simulink model "CryoDetMultiChan_CMB"  (R2016b)
settings: Solver=ode45  StartTime=0.0  StopTime=1000e-6  MaxStep=Tclk/4  RelTol=1e-3
values from neighbouring files (symbols this model uses):
  ds_axi = 16    [setupCryoFPGA_CMB.m]
  Fclk = Fadc    (= 307200000)    [setupCryoFPGA.m]    (also in setupCryoFPGA_CMB.m; setupCryoFPGAorig.m = 312500000)
  notch = tf( [1 a*wNotch/Q wNotch^2], [1 wNotch/Q wNotch^2])    [setupCryoFPGA.m]    (also in setupCryoFPGA_CMB.m; setupCryoFPGAorig.m)
  notch2 = tf( [1 a*wNotch/Q wNotch^2], [1 wNotch/Q wNotch^2])    [setupCryoFPGA.m]    (also in setupCryoFPGA_CMB.m; setupCryoFPGAorig.m)
  notch3 = tf( [1 a*wNotch/Q wNotch^2], [1 wNotch/Q wNotch^2])    [setupCryoFPGA.m]    (also in setupCryoFPGA_CMB.m; setupCryoFPGAorig.m)
  notch4 = tf( [1 a*wNotch/Q wNotch^2], [1 wNotch/Q wNotch^2])    [setupCryoFPGA.m]    (also in setupCryoFPGA_CMB.m; setupCryoFPGAorig.m)
  Tclk = 1/Fclk    (= 3.25520833333e-09)    [setupCryoFPGA.m]    (also in setupCryoFPGA_CMB.m; setupCryoFPGAorig.m = 3.2e-09)
  Ts = 1/Fadc    (= 3.25520833333e-09)    [setupCryoFPGA.m]    (also in setupCryoFPGA_CMB.m; setupCryoFPGAorig.m = 3.2e-09)
undefined symbols (not defined in the file or in its folder): AXI4, i, Lite, xlipgetpartsetting
libraries: xbsIndex_r4 x2077, CryoDetLib x32, hdlsllib x6, simulink x3
(part 4 of 15)

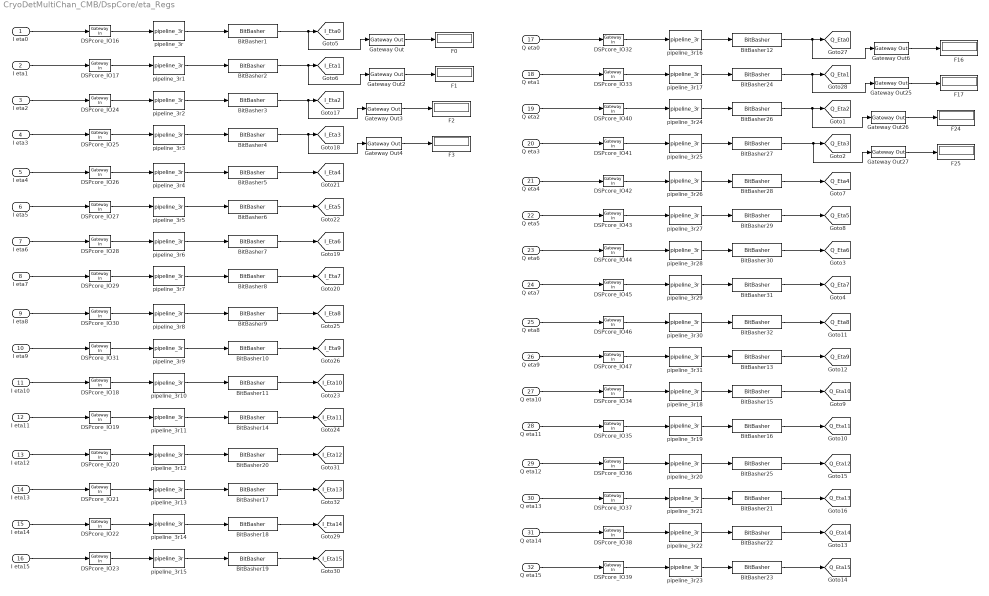
== system CryoDetMultiChan_CMB/DspCore/eta_Regs ==
  "I eta0 " : Inport
  I eta1 : Inport  Port=2
  I eta2 : Inport  Port=3
  I eta3 : Inport  Port=4
  I eta4 : Inport  Port=5
  I eta5 : Inport  Port=6
  I eta6 : Inport  Port=7
  I eta7 : Inport  Port=8
  I eta8 : Inport  Port=9
  I eta9 : Inport  Port=10
  I eta10 : Inport  Port=11
  I eta11 : Inport  Port=12
  I eta12 : Inport  Port=13
  I eta13 : Inport  Port=14
  I eta14 : Inport  Port=15
  I eta15 : Inport  Port=16
  Q eta0 : Inport  Port=17
  Q eta1 : Inport  Port=18
  Q eta2 : Inport  Port=19
  Q eta3 : Inport  Port=20
  Q eta4 : Inport  Port=21
  Q eta5 : Inport  Port=22
  Q eta6 : Inport  Port=23
  Q eta7 : Inport  Port=24
  Q eta8 : Inport  Port=25
  Q eta9 : Inport  Port=26
  Q eta10 : Inport  Port=27
  Q eta11 : Inport  Port=28
  Q eta12 : Inport  Port=29
  Q eta13 : Inport  Port=30
  Q eta14 : Inport  Port=31
  Q eta15 : Inport  Port=32
  BitBasher{1..32} (32 alike) : xbsIndex_r4/BitBasher  bitexpr=a={b[24:0]}  display_expr=on  sr_1=a  arith_type1=Unsigned  bin_pt1=0  sr_2=2  arith_type2=Unsigned  bin_pt2=0  sr_3=3  arith_type3=Unsigned  bin_pt3=0  sr_4=4  arith_type4=Unsigned  bin_pt4=0  dbl_ovrd=off  block_type=bitbasher
  DSPcore_IO16 : xbsIndex_r4/Gateway In  gui_display_data_type=Fixed-point  arith_type="Signed  (2's comp)"  n_bits=32  bin_pt=0  preci_type=Single  exp_width=8  frac_width=24  rows=1  columns=1  quantization=Truncate  overflow=Wrap  period=Tclk*ds_axi  UseAsADC=off  ADCChannel='1'  interface=AXI4-Lite  automatic_assignment=off  address_offset=hex2dec('A00')  intf_name=''  intf_description=''  default_value=0  timing_constraint=None  locs_specified=off  LOCs={}  io_standard={}  inherit_from_input=off  hdl_port=on  dbl_ovrd=off  block_type=gatewayin
  DSPcore_IO17 : xbsIndex_r4/Gateway In  gui_display_data_type=Fixed-point  arith_type="Signed  (2's comp)"  n_bits=32  bin_pt=0  preci_type=Single  exp_width=8  frac_width=24  rows=1  columns=1  quantization=Truncate  overflow=Wrap  period=Tclk*ds_axi  UseAsADC=off  ADCChannel='1'  interface=AXI4-Lite  automatic_assignment=off  address_offset=hex2dec('A08')  intf_name=''  intf_description=''  default_value=0  timing_constraint=None  locs_specified=off  LOCs={}  io_standard={}  inherit_from_input=off  hdl_port=on  dbl_ovrd=off  block_type=gatewayin
  DSPcore_IO18 : xbsIndex_r4/Gateway In  gui_display_data_type=Fixed-point  arith_type="Signed  (2's comp)"  n_bits=32  bin_pt=0  preci_type=Single  exp_width=8  frac_width=24  rows=1  columns=1  quantization=Truncate  overflow=Wrap  period=Tclk*ds_axi  UseAsADC=off  ADCChannel='1'  interface=AXI4-Lite  automatic_assignment=off  address_offset=hex2dec('A50')  intf_name=''  intf_description=''  default_value=0  timing_constraint=None  locs_specified=off  LOCs={}  io_standard={}  inherit_from_input=off  hdl_port=on  dbl_ovrd=off  block_type=gatewayin
  DSPcore_IO19 : xbsIndex_r4/Gateway In  gui_display_data_type=Fixed-point  arith_type="Signed  (2's comp)"  n_bits=32  bin_pt=0  preci_type=Single  exp_width=8  frac_width=24  rows=1  columns=1  quantization=Truncate  overflow=Wrap  period=Tclk*ds_axi  UseAsADC=off  ADCChannel='1'  interface=AXI4-Lite  automatic_assignment=off  address_offset=hex2dec('A58')  intf_name=''  intf_description=''  default_value=0  timing_constraint=None  locs_specified=off  LOCs={}  io_standard={}  inherit_from_input=off  hdl_port=on  dbl_ovrd=off  block_type=gatewayin
  DSPcore_IO20 : xbsIndex_r4/Gateway In  gui_display_data_type=Fixed-point  arith_type="Signed  (2's comp)"  n_bits=32  bin_pt=0  preci_type=Single  exp_width=8  frac_width=24  rows=1  columns=1  quantization=Truncate  overflow=Wrap  period=Tclk*ds_axi  UseAsADC=off  ADCChannel='1'  interface=AXI4-Lite  automatic_assignment=off  address_offset=hex2dec('A60')  intf_name=''  intf_description=''  default_value=0  timing_constraint=None  locs_specified=off  LOCs={}  io_standard={}  inherit_from_input=off  hdl_port=on  dbl_ovrd=off  block_type=gatewayin
  DSPcore_IO21 : xbsIndex_r4/Gateway In  gui_display_data_type=Fixed-point  arith_type="Signed  (2's comp)"  n_bits=32  bin_pt=0  preci_type=Single  exp_width=8  frac_width=24  rows=1  columns=1  quantization=Truncate  overflow=Wrap  period=Tclk*ds_axi  UseAsADC=off  ADCChannel='1'  interface=AXI4-Lite  automatic_assignment=off  address_offset=hex2dec('A68')  intf_name=''  intf_description=''  default_value=0  timing_constraint=None  locs_specified=off  LOCs={}  io_standard={}  inherit_from_input=off  hdl_port=on  dbl_ovrd=off  block_type=gatewayin
  DSPcore_IO22 : xbsIndex_r4/Gateway In  gui_display_data_type=Fixed-point  arith_type="Signed  (2's comp)"  n_bits=32  bin_pt=0  preci_type=Single  exp_width=8  frac_width=24  rows=1  columns=1  quantization=Truncate  overflow=Wrap  period=Tclk*ds_axi  UseAsADC=off  ADCChannel='1'  interface=AXI4-Lite  automatic_assignment=off  address_offset=hex2dec('A70')  intf_name=''  intf_description=''  default_value=0  timing_constraint=None  locs_specified=off  LOCs={}  io_standard={}  inherit_from_input=off  hdl_port=on  dbl_ovrd=off  block_type=gatewayin
  DSPcore_IO23 : xbsIndex_r4/Gateway In  gui_display_data_type=Fixed-point  arith_type="Signed  (2's comp)"  n_bits=32  bin_pt=0  preci_type=Single  exp_width=8  frac_width=24  rows=1  columns=1  quantization=Truncate  overflow=Wrap  period=Tclk*ds_axi  UseAsADC=off  ADCChannel='1'  interface=AXI4-Lite  automatic_assignment=off  address_offset=hex2dec('A78')  intf_name=''  intf_description=''  default_value=0  timing_constraint=None  locs_specified=off  LOCs={}  io_standard={}  inherit_from_input=off  hdl_port=on  dbl_ovrd=off  block_type=gatewayin
  DSPcore_IO24 : xbsIndex_r4/Gateway In  gui_display_data_type=Fixed-point  arith_type="Signed  (2's comp)"  n_bits=32  bin_pt=0  preci_type=Single  exp_width=8  frac_width=24  rows=1  columns=1  quantization=Truncate  overflow=Wrap  period=Tclk*ds_axi  UseAsADC=off  ADCChannel='1'  interface=AXI4-Lite  automatic_assignment=off  address_offset=hex2dec('A10')  intf_name=''  intf_description=''  default_value=0  timing_constraint=None  locs_specified=off  LOCs={}  io_standard={}  inherit_from_input=off  hdl_port=on  dbl_ovrd=off  block_type=gatewayin
  DSPcore_IO25 : xbsIndex_r4/Gateway In  gui_display_data_type=Fixed-point  arith_type="Signed  (2's comp)"  n_bits=32  bin_pt=0  preci_type=Single  exp_width=8  frac_width=24  rows=1  columns=1  quantization=Truncate  overflow=Wrap  period=Tclk*ds_axi  UseAsADC=off  ADCChannel='1'  interface=AXI4-Lite  automatic_assignment=off  address_offset=hex2dec('A18')  intf_name=''  intf_description=''  default_value=0  timing_constraint=None  locs_specified=off  LOCs={}  io_standard={}  inherit_from_input=off  hdl_port=on  dbl_ovrd=off  block_type=gatewayin
  DSPcore_IO26 : xbsIndex_r4/Gateway In  gui_display_data_type=Fixed-point  arith_type="Signed  (2's comp)"  n_bits=32  bin_pt=0  preci_type=Single  exp_width=8  frac_width=24  rows=1  columns=1  quantization=Truncate  overflow=Wrap  period=Tclk*ds_axi  UseAsADC=off  ADCChannel='1'  interface=AXI4-Lite  automatic_assignment=off  address_offset=hex2dec('A20')  intf_name=''  intf_description=''  default_value=0  timing_constraint=None  locs_specified=off  LOCs={}  io_standard={}  inherit_from_input=off  hdl_port=on  dbl_ovrd=off  block_type=gatewayin
  DSPcore_IO27 : xbsIndex_r4/Gateway In  gui_display_data_type=Fixed-point  arith_type="Signed  (2's comp)"  n_bits=32  bin_pt=0  preci_type=Single  exp_width=8  frac_width=24  rows=1  columns=1  quantization=Truncate  overflow=Wrap  period=Tclk*ds_axi  UseAsADC=off  ADCChannel='1'  interface=AXI4-Lite  automatic_assignment=off  address_offset=hex2dec('A28')  intf_name=''  intf_description=''  default_value=0  timing_constraint=None  locs_specified=off  LOCs={}  io_standard={}  inherit_from_input=off  hdl_port=on  dbl_ovrd=off  block_type=gatewayin
  DSPcore_IO28 : xbsIndex_r4/Gateway In  gui_display_data_type=Fixed-point  arith_type="Signed  (2's comp)"  n_bits=32  bin_pt=0  preci_type=Single  exp_width=8  frac_width=24  rows=1  columns=1  quantization=Truncate  overflow=Wrap  period=Tclk*ds_axi  UseAsADC=off  ADCChannel='1'  interface=AXI4-Lite  automatic_assignment=off  address_offset=hex2dec('A30')  intf_name=''  intf_description=''  default_value=0  timing_constraint=None  locs_specified=off  LOCs={}  io_standard={}  inherit_from_input=off  hdl_port=on  dbl_ovrd=off  block_type=gatewayin
  DSPcore_IO29 : xbsIndex_r4/Gateway In  gui_display_data_type=Fixed-point  arith_type="Signed  (2's comp)"  n_bits=32  bin_pt=0  preci_type=Single  exp_width=8  frac_width=24  rows=1  columns=1  quantization=Truncate  overflow=Wrap  period=Tclk*ds_axi  UseAsADC=off  ADCChannel='1'  interface=AXI4-Lite  automatic_assignment=off  address_offset=hex2dec('A38')  intf_name=''  intf_description=''  default_value=0  timing_constraint=None  locs_specified=off  LOCs={}  io_standard={}  inherit_from_input=off  hdl_port=on  dbl_ovrd=off  block_type=gatewayin
  DSPcore_IO30 : xbsIndex_r4/Gateway In  gui_display_data_type=Fixed-point  arith_type="Signed  (2's comp)"  n_bits=32  bin_pt=0  preci_type=Single  exp_width=8  frac_width=24  rows=1  columns=1  quantization=Truncate  overflow=Wrap  period=Tclk*ds_axi  UseAsADC=off  ADCChannel='1'  interface=AXI4-Lite  automatic_assignment=off  address_offset=hex2dec('A40')  intf_name=''  intf_description=''  default_value=0  timing_constraint=None  locs_specified=off  LOCs={}  io_standard={}  inherit_from_input=off  hdl_port=on  dbl_ovrd=off  block_type=gatewayin
  DSPcore_IO31 : xbsIndex_r4/Gateway In  gui_display_data_type=Fixed-point  arith_type="Signed  (2's comp)"  n_bits=32  bin_pt=0  preci_type=Single  exp_width=8  frac_width=24  rows=1  columns=1  quantization=Truncate  overflow=Wrap  period=Tclk*ds_axi  UseAsADC=off  ADCChannel='1'  interface=AXI4-Lite  automatic_assignment=off  address_offset=hex2dec('A48')  intf_name=''  intf_description=''  default_value=0  timing_constraint=None  locs_specified=off  LOCs={}  io_standard={}  inherit_from_input=off  hdl_port=on  dbl_ovrd=off  block_type=gatewayin
  DSPcore_IO32 : xbsIndex_r4/Gateway In  gui_display_data_type=Fixed-point  arith_type="Signed  (2's comp)"  n_bits=32  bin_pt=0  preci_type=Single  exp_width=8  frac_width=24  rows=1  columns=1  quantization=Truncate  overflow=Wrap  period=Tclk*ds_axi  UseAsADC=off  ADCChannel='1'  interface=AXI4-Lite  automatic_assignment=off  address_offset=hex2dec('A04')  intf_name=''  intf_description=''  default_value=0  timing_constraint=None  locs_specified=off  LOCs={}  io_standard={}  inherit_from_input=off  hdl_port=on  dbl_ovrd=off  block_type=gatewayin
  DSPcore_IO33 : xbsIndex_r4/Gateway In  gui_display_data_type=Fixed-point  arith_type="Signed  (2's comp)"  n_bits=32  bin_pt=0  preci_type=Single  exp_width=8  frac_width=24  rows=1  columns=1  quantization=Truncate  overflow=Wrap  period=Tclk*ds_axi  UseAsADC=off  ADCChannel='1'  interface=AXI4-Lite  automatic_assignment=off  address_offset=hex2dec('A0C')  intf_name=''  intf_description=''  default_value=0  timing_constraint=None  locs_specified=off  LOCs={}  io_standard={}  inherit_from_input=off  hdl_port=on  dbl_ovrd=off  block_type=gatewayin
  DSPcore_IO34 : xbsIndex_r4/Gateway In  gui_display_data_type=Fixed-point  arith_type="Signed  (2's comp)"  n_bits=32  bin_pt=0  preci_type=Single  exp_width=8  frac_width=24  rows=1  columns=1  quantization=Truncate  overflow=Wrap  period=Tclk*ds_axi  UseAsADC=off  ADCChannel='1'  interface=AXI4-Lite  automatic_assignment=off  address_offset=hex2dec('A54')  intf_name=''  intf_description=''  default_value=0  timing_constraint=None  locs_specified=off  LOCs={}  io_standard={}  inherit_from_input=off  hdl_port=on  dbl_ovrd=off  block_type=gatewayin
  DSPcore_IO35 : xbsIndex_r4/Gateway In  gui_display_data_type=Fixed-point  arith_type="Signed  (2's comp)"  n_bits=32  bin_pt=0  preci_type=Single  exp_width=8  frac_width=24  rows=1  columns=1  quantization=Truncate  overflow=Wrap  period=Tclk*ds_axi  UseAsADC=off  ADCChannel='1'  interface=AXI4-Lite  automatic_assignment=off  address_offset=hex2dec('A5C')  intf_name=''  intf_description=''  default_value=0  timing_constraint=None  locs_specified=off  LOCs={}  io_standard={}  inherit_from_input=off  hdl_port=on  dbl_ovrd=off  block_type=gatewayin
  DSPcore_IO36 : xbsIndex_r4/Gateway In  gui_display_data_type=Fixed-point  arith_type="Signed  (2's comp)"  n_bits=32  bin_pt=0  preci_type=Single  exp_width=8  frac_width=24  rows=1  columns=1  quantization=Truncate  overflow=Wrap  period=Tclk*ds_axi  UseAsADC=off  ADCChannel='1'  interface=AXI4-Lite  automatic_assignment=off  address_offset=hex2dec('A64')  intf_name=''  intf_description=''  default_value=0  timing_constraint=None  locs_specified=off  LOCs={}  io_standard={}  inherit_from_input=off  hdl_port=on  dbl_ovrd=off  block_type=gatewayin
  DSPcore_IO37 : xbsIndex_r4/Gateway In  gui_display_data_type=Fixed-point  arith_type="Signed  (2's comp)"  n_bits=32  bin_pt=0  preci_type=Single  exp_width=8  frac_width=24  rows=1  columns=1  quantization=Truncate  overflow=Wrap  period=Tclk*ds_axi  UseAsADC=off  ADCChannel='1'  interface=AXI4-Lite  automatic_assignment=off  address_offset=hex2dec('A6C')  intf_name=''  intf_description=''  default_value=0  timing_constraint=None  locs_specified=off  LOCs={}  io_standard={}  inherit_from_input=off  hdl_port=on  dbl_ovrd=off  block_type=gatewayin
  DSPcore_IO38 : xbsIndex_r4/Gateway In  gui_display_data_type=Fixed-point  arith_type="Signed  (2's comp)"  n_bits=32  bin_pt=0  preci_type=Single  exp_width=8  frac_width=24  rows=1  columns=1  quantization=Truncate  overflow=Wrap  period=Tclk*ds_axi  UseAsADC=off  ADCChannel='1'  interface=AXI4-Lite  automatic_assignment=off  address_offset=hex2dec('A74')  intf_name=''  intf_description=''  default_value=0  timing_constraint=None  locs_specified=off  LOCs={}  io_standard={}  inherit_from_input=off  hdl_port=on  dbl_ovrd=off  block_type=gatewayin
  DSPcore_IO39 : xbsIndex_r4/Gateway In  gui_display_data_type=Fixed-point  arith_type="Signed  (2's comp)"  n_bits=32  bin_pt=0  preci_type=Single  exp_width=8  frac_width=24  rows=1  columns=1  quantization=Truncate  overflow=Wrap  period=Tclk*ds_axi  UseAsADC=off  ADCChannel='1'  interface=AXI4-Lite  automatic_assignment=off  address_offset=hex2dec('A7C')  intf_name=''  intf_description=''  default_value=0  timing_constraint=None  locs_specified=off  LOCs={}  io_standard={}  inherit_from_input=off  hdl_port=on  dbl_ovrd=off  block_type=gatewayin
  DSPcore_IO40 : xbsIndex_r4/Gateway In  gui_display_data_type=Fixed-point  arith_type="Signed  (2's comp)"  n_bits=32  bin_pt=0  preci_type=Single  exp_width=8  frac_width=24  rows=1  columns=1  quantization=Truncate  overflow=Wrap  period=Tclk*ds_axi  UseAsADC=off  ADCChannel='1'  interface=AXI4-Lite  automatic_assignment=off  address_offset=hex2dec('A14')  intf_name=''  intf_description=''  default_value=0  timing_constraint=None  locs_specified=off  LOCs={}  io_standard={}  inherit_from_input=off  hdl_port=on  dbl_ovrd=off  block_type=gatewayin
  DSPcore_IO41 : xbsIndex_r4/Gateway In  gui_display_data_type=Fixed-point  arith_type="Signed  (2's comp)"  n_bits=32  bin_pt=0  preci_type=Single  exp_width=8  frac_width=24  rows=1  columns=1  quantization=Truncate  overflow=Wrap  period=Tclk*ds_axi  UseAsADC=off  ADCChannel='1'  interface=AXI4-Lite  automatic_assignment=off  address_offset=hex2dec('A1C')  intf_name=''  intf_description=''  default_value=0  timing_constraint=None  locs_specified=off  LOCs={}  io_standard={}  inherit_from_input=off  hdl_port=on  dbl_ovrd=off  block_type=gatewayin
  DSPcore_IO42 : xbsIndex_r4/Gateway In  gui_display_data_type=Fixed-point  arith_type="Signed  (2's comp)"  n_bits=32  bin_pt=0  preci_type=Single  exp_width=8  frac_width=24  rows=1  columns=1  quantization=Truncate  overflow=Wrap  period=Tclk*ds_axi  UseAsADC=off  ADCChannel='1'  interface=AXI4-Lite  automatic_assignment=off  address_offset=hex2dec('A24')  intf_name=''  intf_description=''  default_value=0  timing_constraint=None  locs_specified=off  LOCs={}  io_standard={}  inherit_from_input=off  hdl_port=on  dbl_ovrd=off  block_type=gatewayin
  DSPcore_IO43 : xbsIndex_r4/Gateway In  gui_display_data_type=Fixed-point  arith_type="Signed  (2's comp)"  n_bits=32  bin_pt=0  preci_type=Single  exp_width=8  frac_width=24  rows=1  columns=1  quantization=Truncate  overflow=Wrap  period=Tclk*ds_axi  UseAsADC=off  ADCChannel='1'  interface=AXI4-Lite  automatic_assignment=off  address_offset=hex2dec('A2C')  intf_name=''  intf_description=''  default_value=0  timing_constraint=None  locs_specified=off  LOCs={}  io_standard={}  inherit_from_input=off  hdl_port=on  dbl_ovrd=off  block_type=gatewayin
  DSPcore_IO44 : xbsIndex_r4/Gateway In  gui_display_data_type=Fixed-point  arith_type="Signed  (2's comp)"  n_bits=32  bin_pt=0  preci_type=Single  exp_width=8  frac_width=24  rows=1  columns=1  quantization=Truncate  overflow=Wrap  period=Tclk*ds_axi  UseAsADC=off  ADCChannel='1'  interface=AXI4-Lite  automatic_assignment=off  address_offset=hex2dec('A34')  intf_name=''  intf_description=''  default_value=0  timing_constraint=None  locs_specified=off  LOCs={}  io_standard={}  inherit_from_input=off  hdl_port=on  dbl_ovrd=off  block_type=gatewayin
  DSPcore_IO45 : xbsIndex_r4/Gateway In  gui_display_data_type=Fixed-point  arith_type="Signed  (2's comp)"  n_bits=32  bin_pt=0  preci_type=Single  exp_width=8  frac_width=24  rows=1  columns=1  quantization=Truncate  overflow=Wrap  period=Tclk*ds_axi  UseAsADC=off  ADCChannel='1'  interface=AXI4-Lite  automatic_assignment=off  address_offset=hex2dec('A3C')  intf_name=''  intf_description=''  default_value=0  timing_constraint=None  locs_specified=off  LOCs={}  io_standard={}  inherit_from_input=off  hdl_port=on  dbl_ovrd=off  block_type=gatewayin
  DSPcore_IO46 : xbsIndex_r4/Gateway In  gui_display_data_type=Fixed-point  arith_type="Signed  (2's comp)"  n_bits=32  bin_pt=0  preci_type=Single  exp_width=8  frac_width=24  rows=1  columns=1  quantization=Truncate  overflow=Wrap  period=Tclk*ds_axi  UseAsADC=off  ADCChannel='1'  interface=AXI4-Lite  automatic_assignment=off  address_offset=hex2dec('A44')  intf_name=''  intf_description=''  default_value=0  timing_constraint=None  locs_specified=off  LOCs={}  io_standard={}  inherit_from_input=off  hdl_port=on  dbl_ovrd=off  block_type=gatewayin
  DSPcore_IO47 : xbsIndex_r4/Gateway In  gui_display_data_type=Fixed-point  arith_type="Signed  (2's comp)"  n_bits=32  bin_pt=0  preci_type=Single  exp_width=8  frac_width=24  rows=1  columns=1  quantization=Truncate  overflow=Wrap  period=Tclk*ds_axi  UseAsADC=off  ADCChannel='1'  interface=AXI4-Lite  automatic_assignment=off  address_offset=hex2dec('A4C')  intf_name=''  intf_description=''  default_value=0  timing_constraint=None  locs_specified=off  LOCs={}  io_standard={}  inherit_from_input=off  hdl_port=on  dbl_ovrd=off  block_type=gatewayin
  F{0..3,16..17,24..25} (8 alike) : Display
  Gateway Out{,2..4,6,25..27} (8 alike) : xbsIndex_r4/Gateway Out  inherit_from_input=on  hdl_port=off  rows=1  columns=1  UseAsDAC=off  DACChannel='1'  interface=None  automatic_assignment=on  address_offset=hex2dec('00')  intf_name=''  intf_description=''  timing_constraint=None  locs_specified=off  LOCs={}  io_standard={}  block_type=gatewayout
  pipeline_3r{,1..31} (32 alike) : CryoDetLib/pipeline_3r
  tag scope: I_Eta0=global, I_Eta10=global, I_Eta11=global, I_Eta12=global, I_Eta13=global, I_Eta14=global, I_Eta15=global, I_Eta1=global, I_Eta2=global, I_Eta3=global, I_Eta4=global, I_Eta5=global, I_Eta6=global, I_Eta7=global, I_Eta8=global, I_Eta9=global, Q_Eta0=global, Q_Eta10=global, Q_Eta11=global, Q_Eta12=global, Q_Eta13=global, Q_Eta14=global, Q_Eta15=global, Q_Eta1=global, Q_Eta2=global, Q_Eta3=global, Q_Eta4=global, Q_Eta5=global, Q_Eta6=global, Q_Eta7=global, Q_Eta8=global, Q_Eta9=global
  wires:
  I eta14/1 -> DSPcore_IO22/1
  BitBasher5/1 -> [I_Eta4]
  DSPcore_IO26/1 -> pipeline_3r4/1
  BitBasher17/1 -> [I_Eta13]
  I eta13/1 -> DSPcore_IO21/1
  DSPcore_IO27/1 -> pipeline_3r5/1
  I eta15/1 -> DSPcore_IO23/1
  BitBasher11/1 -> [I_Eta10]
  I eta7/1 -> DSPcore_IO29/1
  I eta11/1 -> DSPcore_IO19/1
  I eta9/1 -> DSPcore_IO31/1
  Gateway Out4/1 -> F3/1
  BitBasher4/1 -> [I_Eta3], Gateway Out4/1
  I eta5/1 -> DSPcore_IO27/1
  DSPcore_IO23/1 -> pipeline_3r15/1
  DSPcore_IO21/1 -> pipeline_3r13/1
  DSPcore_IO31/1 -> pipeline_3r9/1
  BitBasher6/1 -> [I_Eta5]
  I eta8/1 -> DSPcore_IO30/1
  DSPcore_IO20/1 -> pipeline_3r12/1
  BitBasher20/1 -> [I_Eta12]
  DSPcore_IO25/1 -> pipeline_3r3/1
  I eta4/1 -> DSPcore_IO26/1
  Gateway Out2/1 -> F1/1
  BitBasher2/1 -> [I_Eta1], Gateway Out2/1
  DSPcore_IO30/1 -> pipeline_3r8/1
  BitBasher14/1 -> [I_Eta11]
  BitBasher19/1 -> [I_Eta15]
  I eta10/1 -> DSPcore_IO18/1
  BitBasher10/1 -> [I_Eta9]
  DSPcore_IO19/1 -> pipeline_3r11/1
  DSPcore_IO24/1 -> pipeline_3r2/1
  I eta2/1 -> DSPcore_IO24/1
  Gateway Out3/1 -> F2/1
  BitBasher3/1 -> [I_Eta2], Gateway Out3/1
  DSPcore_IO22/1 -> pipeline_3r14/1
  DSPcore_IO17/1 -> pipeline_3r1/1
  I eta1/1 -> DSPcore_IO17/1
  BitBasher9/1 -> [I_Eta8]
  DSPcore_IO29/1 -> pipeline_3r7/1
  BitBasher18/1 -> [I_Eta14]
  DSPcore_IO18/1 -> pipeline_3r10/1
  I eta6/1 -> DSPcore_IO28/1
  I eta3/1 -> DSPcore_IO25/1
  "I eta0 "/1 -> DSPcore_IO16/1
  Gateway Out/1 -> F0/1
  BitBasher1/1 -> [I_Eta0], Gateway Out/1
  DSPcore_IO16/1 -> pipeline_3r/1
  pipeline_3r/1 -> BitBasher1/1
  BitBasher7/1 -> [I_Eta6]
  BitBasher8/1 -> [I_Eta7]
  I eta12/1 -> DSPcore_IO20/1
  DSPcore_IO28/1 -> pipeline_3r6/1
  Q eta14/1 -> DSPcore_IO38/1
  BitBasher28/1 -> [Q_Eta4]
  DSPcore_IO42/1 -> pipeline_3r26/1
  BitBasher21/1 -> [Q_Eta13]
  Q eta13/1 -> DSPcore_IO37/1
  DSPcore_IO43/1 -> pipeline_3r27/1
  Q eta15/1 -> DSPcore_IO39/1
  BitBasher15/1 -> [Q_Eta10]
  Q eta7/1 -> DSPcore_IO45/1
  Q eta11/1 -> DSPcore_IO35/1
  Q eta9/1 -> DSPcore_IO47/1
  Gateway Out27/1 -> F25/1
  BitBasher27/1 -> [Q_Eta3], Gateway Out27/1
  Q eta5/1 -> DSPcore_IO43/1
  DSPcore_IO39/1 -> pipeline_3r23/1
  DSPcore_IO37/1 -> pipeline_3r21/1
  DSPcore_IO47/1 -> pipeline_3r31/1
  BitBasher29/1 -> [Q_Eta5]
  Q eta8/1 -> DSPcore_IO46/1
  DSPcore_IO36/1 -> pipeline_3r20/1
  BitBasher25/1 -> [Q_Eta12]
  DSPcore_IO41/1 -> pipeline_3r25/1
  Q eta4/1 -> DSPcore_IO42/1
  Gateway Out25/1 -> F17/1
  BitBasher24/1 -> [Q_Eta1], Gateway Out25/1
  DSPcore_IO46/1 -> pipeline_3r30/1
  BitBasher16/1 -> [Q_Eta11]
  BitBasher23/1 -> [Q_Eta15]
  Q eta10/1 -> DSPcore_IO34/1
  BitBasher13/1 -> [Q_Eta9]
  DSPcore_IO35/1 -> pipeline_3r19/1
  DSPcore_IO40/1 -> pipeline_3r24/1
  Q eta2/1 -> DSPcore_IO40/1
  Gateway Out26/1 -> F24/1
  BitBasher26/1 -> [Q_Eta2], Gateway Out26/1
  DSPcore_IO38/1 -> pipeline_3r22/1
  DSPcore_IO33/1 -> pipeline_3r17/1
  Q eta1/1 -> DSPcore_IO33/1
  BitBasher32/1 -> [Q_Eta8]
  DSPcore_IO45/1 -> pipeline_3r29/1
  BitBasher22/1 -> [Q_Eta14]
  DSPcore_IO34/1 -> pipeline_3r18/1
  Q eta6/1 -> DSPcore_IO44/1
  Q eta3/1 -> DSPcore_IO41/1
  Q eta0/1 -> DSPcore_IO32/1
  Gateway Out6/1 -> F16/1
  BitBasher12/1 -> [Q_Eta0], Gateway Out6/1
  DSPcore_IO32/1 -> pipeline_3r16/1
  BitBasher30/1 -> [Q_Eta6]
  BitBasher31/1 -> [Q_Eta7]
  Q eta12/1 -> DSPcore_IO36/1
  DSPcore_IO44/1 -> pipeline_3r28/1
  pipeline_3r1/1 -> BitBasher2/1
  pipeline_3r2/1 -> BitBasher3/1
  pipeline_3r3/1 -> BitBasher4/1
  pipeline_3r6/1 -> BitBasher7/1
  pipeline_3r7/1 -> BitBasher8/1
  pipeline_3r5/1 -> BitBasher6/1
  pipeline_3r4/1 -> BitBasher5/1
  pipeline_3r8/1 -> BitBasher9/1
  pipeline_3r10/1 -> BitBasher11/1
  pipeline_3r11/1 -> BitBasher14/1
  pipeline_3r9/1 -> BitBasher10/1
  pipeline_3r15/1 -> BitBasher19/1
  pipeline_3r13/1 -> BitBasher17/1
  pipeline_3r14/1 -> BitBasher18/1
  pipeline_3r12/1 -> BitBasher20/1
  pipeline_3r16/1 -> BitBasher12/1
  pipeline_3r19/1 -> BitBasher16/1
  pipeline_3r26/1 -> BitBasher28/1
  pipeline_3r23/1 -> BitBasher23/1
  pipeline_3r24/1 -> BitBasher26/1
  pipeline_3r28/1 -> BitBasher30/1
  pipeline_3r20/1 -> BitBasher25/1
  pipeline_3r22/1 -> BitBasher22/1
  pipeline_3r25/1 -> BitBasher27/1
  pipeline_3r30/1 -> BitBasher32/1
  pipeline_3r17/1 -> BitBasher24/1
  pipeline_3r18/1 -> BitBasher15/1
  pipeline_3r27/1 -> BitBasher29/1
  pipeline_3r21/1 -> BitBasher21/1
  pipeline_3r31/1 -> BitBasher13/1
  pipeline_3r29/1 -> BitBasher31/1

== system CryoDetMultiChan_CMB/complex Notch0/imNotch ==
  note: Notch Filter with center angular frequency w, finite Q, and depth -26 dB
  In : Inport
  w0 : Inport  Port=2
  1/Q : Inport  Port=3
  Gain : Gain  Gain=.90
  Integrator1 : Integrator
  Integrator4 : Integrator
  Mult : Product
  Product : Product
  Product1 : Product
  Sum1 : Sum  Inputs=++|
  Sum2 : Sum  Inputs=|+-
  Sum3 : Sum  Inputs=-+|
  outt : Outport
  wires:
  w0/1 -> Product1/1, Product/1
  Integrator1/1 -> Product/2
  Product/1 -> Mult/1, Integrator4/1
  Integrator4/1 -> Product1/2
  1/Q/1 -> Mult/2
  Sum2/1 -> Integrator1/1
  In/1 -> Sum3/2, Sum2/1
  Sum1/1 -> Sum2/2
  Product1/1 -> Sum1/2
  Mult/1 -> Gain/1, Sum1/1
  Sum3/1 -> outt/1
  Gain/1 -> Sum3/1

== system CryoDetMultiChan_CMB/complex Notch0/reNotch ==
  note: Notch Filter with center angular frequency w, finite Q, and depth -26 dB
  In : Inport
  w0 : Inport  Port=2
  1/Q : Inport  Port=3
  Gain : Gain  Gain=.90
  Integrator1 : Integrator
  Integrator4 : Integrator
  Mult : Product
  Product : Product
  Product1 : Product
  Sum1 : Sum  Inputs=++|
  Sum2 : Sum  Inputs=|+-
  Sum3 : Sum  Inputs=-+|
  outt : Outport
  wires:
  w0/1 -> Product1/1, Product/1
  Integrator1/1 -> Product/2
  Product/1 -> Mult/1, Integrator4/1
  Integrator4/1 -> Product1/2
  1/Q/1 -> Mult/2
  Sum2/1 -> Integrator1/1
  In/1 -> Sum3/2, Sum2/1
  Sum1/1 -> Sum2/2
  Product1/1 -> Sum1/2
  Mult/1 -> Gain/1, Sum1/1
  Sum3/1 -> outt/1
  Gain/1 -> Sum3/1

== system CryoDetMultiChan_CMB/complex Notch1/imNotch ==
  note: Notch Filter with center angular frequency w, finite Q, and depth -26 dB
  In : Inport
  w0 : Inport  Port=2
  1/Q : Inport  Port=3
  Gain : Gain  Gain=.90
  Integrator1 : Integrator
  Integrator4 : Integrator
  Mult : Product
  Product : Product
  Product1 : Product
  Sum1 : Sum  Inputs=++|
  Sum2 : Sum  Inputs=|+-
  Sum3 : Sum  Inputs=-+|
  outt : Outport
  wires:
  w0/1 -> Product1/1, Product/1
  Integrator1/1 -> Product/2
  Product/1 -> Mult/1, Integrator4/1
  Integrator4/1 -> Product1/2
  1/Q/1 -> Mult/2
  Sum2/1 -> Integrator1/1
  In/1 -> Sum3/2, Sum2/1
  Sum1/1 -> Sum2/2
  Product1/1 -> Sum1/2
  Mult/1 -> Gain/1, Sum1/1
  Sum3/1 -> outt/1
  Gain/1 -> Sum3/1

== system CryoDetMultiChan_CMB/complex Notch1/reNotch ==
  note: Notch Filter with center angular frequency w, finite Q, and depth -26 dB
  In : Inport
  w0 : Inport  Port=2
  1/Q : Inport  Port=3
  Gain : Gain  Gain=.90
  Integrator1 : Integrator
  Integrator4 : Integrator
  Mult : Product
  Product : Product
  Product1 : Product
  Sum1 : Sum  Inputs=++|
  Sum2 : Sum  Inputs=|+-
  Sum3 : Sum  Inputs=-+|
  outt : Outport
  wires:
  w0/1 -> Product1/1, Product/1
  Integrator1/1 -> Product/2
  Product/1 -> Mult/1, Integrator4/1
  Integrator4/1 -> Product1/2
  1/Q/1 -> Mult/2
  Sum2/1 -> Integrator1/1
  In/1 -> Sum3/2, Sum2/1
  Sum1/1 -> Sum2/2
  Product1/1 -> Sum1/2
  Mult/1 -> Gain/1, Sum1/1
  Sum3/1 -> outt/1
  Gain/1 -> Sum3/1

== system CryoDetMultiChan_CMB/DspCore/FTA_Ch0/ADC_IQ_Swap ==
  note: BAND 1 Input
  note: I & Q Swap Logic
      |
      | Added b/c I'm not sure how the ADC
      | actually maps the I & Q data onto the 32-b word
      | Once we work this out, it can be hard-wired
  Swap_en : Inport
  ADC_in : Inport  Port=2
  BitBasher : xbsIndex_r4/BitBasher  bitexpr=|  display_expr=off  sr_1=I  arith_type1="Signed  (2's comp)"  bin_pt1=15  sr_2=Q  arith_type2="Signed  (2's comp)"  bin_pt2=15  sr_3=3  arith_type3=Unsigned  bin_pt3=0  sr_4=4  arith_type4=Unsigned  bin_pt4=0  dbl_ovrd=off  block_type=bitbasher
      | I = {a[15:0]}
      | Q = {a[31:16]}
  Mux8 : xbsIndex_r4/Mux  inputs=2  en=off  latency=1  precision=Full  arith_type=Unsigned  n_bits=16  bin_pt=14  quantization=Truncate  overflow=Wrap  dbl_ovrd=off  block_type=mux
  Mux9 : xbsIndex_r4/Mux  inputs=2  en=off  latency=1  precision=Full  arith_type=Unsigned  n_bits=16  bin_pt=14  quantization=Truncate  overflow=Wrap  dbl_ovrd=off  block_type=mux
  ADC_I_out : Outport
  ADC_Q_out : Outport  Port=2
  wires:
  Mux8/1 -> ADC_I_out/1
  ADC_in/1 -> BitBasher/1
  Swap_en/1 -> Mux8/1, Mux9/1
  BitBasher/1 -> Mux9/3, Mux8/2
  BitBasher/2 -> Mux9/2, Mux8/3
  Mux9/1 -> ADC_Q_out/1

== system CryoDetMultiChan_CMB/DspCore/FTA_Ch0/DAC_Output_Fmt ==
  In1 : Inport
  BitBasher : xbsIndex_r4/BitBasher  bitexpr=|  display_expr=off  sr_1=DAC_Q  arith_type1=Unsigned  bin_pt1=0  sr_2=DAC_I  arith_type2=Unsigned  bin_pt2=0  sr_3=3  arith_type3=Unsigned  bin_pt3=0  sr_4=4  arith_type4=Unsigned  bin_pt4=0  dbl_ovrd=off  block_type=bitbasher
      | DAC_Q={Q[15:0],Qp[15:0]}
      | DAC_I={I[15:0],Ip[15:0]}
  Bus Selector : BusSelector  OutputSignals=DAC_out_Q,DAC_out_I,DAC_out_Qp,DAC_out_Ip
  Out_Q : Outport
  Out_I : Outport  Port=2
  wires:
  BitBasher/2 -> Out_I/1
  Bus Selector/2 -> BitBasher/2  "<DAC_out_I>"
  In1/1 -> Bus Selector/1
  Bus Selector/1 -> BitBasher/1  "<DAC_out_Q>"
  BitBasher/1 -> Out_Q/1
  Bus Selector/4 -> BitBasher/4  "<DAC_out_Ip>"
  Bus Selector/3 -> BitBasher/3  "<DAC_out_Qp>"

== system CryoDetMultiChan_CMB/DspCore/FTA_Ch0/RF switch ==
  note: Enable/disable RF
  note: To DAC
  note: From tone generators
  note: To Ref
  In1 : Inport
  Bus Creator : BusCreator  Inputs=4
  Bus Creator1 : BusCreator  Inputs=2
  Bus Selector : BusSelector  OutputSignals=Q sum,I sum,Qp sum,Ip sum
  Constant2 : xbsIndex_r4/Constant  const=0  gui_display_data_type=Fixed-point  arith_type=Signed (2's comp)  n_bits=16  bin_pt=15  preci_type=Single  exp_width=8  frac_width=24  explicit_period=off  period=1  equ=P=C  opselect=C  inp2=PCIN>>17  opr=+  inp1=P  carry=CIN  dbl_ovrd=off  block_type=constant
  Mux{1..4} (4 alike) : xbsIndex_r4/Mux  inputs=2  en=off  latency=1  precision=User Defined  arith_type="Signed  (2's comp)"  n_bits=16  bin_pt=15  quantization=Truncate  overflow=Flag as error  dbl_ovrd=off  block_type=mux
  RF switch scope : Scope  NumInputPorts=5
  to_DAC : Outport
  to_REF : Outport  Port=2
  wires:
  [RFen] -> RF switch scope/1, Mux3/1, Mux4/1, Mux1/1, Mux2/1
  Constant2/1 -> Mux4/2, Mux3/2, Mux1/2, Mux2/2
  Bus Creator/1 -> to_DAC/1
  In1/1 -> Bus Selector/1
  Mux2/1 -> Bus Creator1/1, Bus Creator/1  "DAC_Q"
  Mux1/1 -> Bus Creator1/2, Bus Creator/2, RF switch scope/4  "DAC_I"
  Mux4/1 -> Bus Creator/3  "DAC_Qp"
  Mux3/1 -> RF switch scope/5, Bus Creator/4  "DAC_Ip"
  Bus Selector/1 -> Mux2/3  "<Q sum>"
  Bus Selector/2 -> RF switch scope/2, Mux1/3  "<I sum>"
  Bus Selector/3 -> Mux4/3  "<Qp sum>"
  Bus Selector/4 -> RF switch scope/3, Mux3/3  "<Ip sum>"
  Bus Creator1/1 -> to_REF/1

== system CryoDetMultiChan_CMB/DspCore/FTA_Ch0/Ref Delay ==
  note: Delays DAC output data used as Reference for input signal
      | Delay is to compensate for delay of DAC (big), up/downconverter, cable plant, cryostat etc.
      | This is to prevent too much delay mismatch from winding up phase vs. frequency of S21's of sidebands wrt to central line
  In1 : Inport
  Addressable Shift Register : xbsIndex_r4/Addressable Shift Register  infer_latency=on  depth=2  initVector=[0]  en=off  use_behavioral_HDL=on  Optimization=Resource  dbl_ovrd=off  block_type=addrsr
      settings: infoedit="Delay of configurable length.  Any element in the delay line can be addressed and driven onto the output port.<br><br>Hardware notes: Generates fast, compact FIFO-style shift registers or delay lines using SRL16/SRL32 mode of the slice LUTs"
  Addressable Shift Register1 : xbsIndex_r4/Addressable Shift Register  infer_latency=on  depth=2  initVector=[0]  en=off  use_behavioral_HDL=on  Optimization=Resource  dbl_ovrd=off  block_type=addrsr
      settings: infoedit="Delay of configurable length.  Any element in the delay line can be addressed and driven onto the output port.<br><br>Hardware notes: Generates fast, compact FIFO-style shift registers or delay lines using SRL16/SRL32 mode of the slice LUTs"
  Bus Selector : BusSelector  OutputSignals=DAC_Q,DAC_I
  Display : Display
      settings: Decimation=128
  Gateway Out : xbsIndex_r4/Gateway Out  inherit_from_input=off  hdl_port=off  rows=1  columns=1  UseAsDAC=off  DACChannel='1'  interface=None  automatic_assignment=on  address_offset=hex2dec('00')  intf_name=''  intf_description=''  timing_constraint=None  locs_specified=off  LOCs={}  io_standard={}  block_type=gatewayout
  Out_Q : Outport
  Out_I : Outport  Port=2
  wires:
  In1/1 -> Bus Selector/1
  Bus Selector/2 -> Addressable Shift Register1/1  "<DAC_I>"
  Bus Selector/1 -> Addressable Shift Register/1  "<DAC_Q>"
  Gateway Out/1 -> Display/1
  Addressable Shift Register/1 -> Out_Q/1
  Addressable Shift Register1/1 -> Out_I/1
  [refDel] -> Addressable Shift Register1/2, Addressable Shift Register/2, Gateway Out/1

== system CryoDetMultiChan_CMB/DspCore/FTA_Ch0/SixteenLineUDC 0 ==
  note: Intentionally swapping REF I & Q
  note: SixteenLineUDC(n)
      |
      | Implelents the Up *and* Down Conversion for each Resonator Line/Channel
      | One Block implements one U/D converter pair
      | The counter use used to syncronize the internal CIC filter reset operation to allow the data to be interleaved
      | The MUX16x4 block does the actual time-domain interleaving operation
      | The DC Decimate block does a further decimate and filtering operation on the ADC and Reference signals before sending them downstream for furhter processing
      | The DAC SUM block individually sums the I & Q components of the upconverted signals (4 individual sum streams from the DAC & DAC + phi signals) before they are forwarded downstream.
  ADC_I_in : Inport
  ADC_Q_in : Inport  Port=2
  REF_I_in1 : Inport  Port=3
  REF_Q_in1 : Inport  Port=4
  BDC scope : Scope  NumInputPorts=2
  Constant : xbsIndex_r4/Constant  const=0  gui_display_data_type=Fixed-point  arith_type=Unsigned  n_bits=5  bin_pt=0  preci_type=Single  exp_width=8  frac_width=24  explicit_period=off  period=1  equ=P=C  opselect=C  inp2=PCIN>>17  opr=+  inp1=P  carry=CIN  dbl_ovrd=off  block_type=constant
  Constant1 : xbsIndex_r4/Constant  const=1  gui_display_data_type=Fixed-point  arith_type=Unsigned  n_bits=5  bin_pt=0  preci_type=Single  exp_width=8  frac_width=24  explicit_period=off  period=1  equ=P=C  opselect=C  inp2=PCIN>>17  opr=+  inp1=P  carry=CIN  dbl_ovrd=off  block_type=constant
  Constant10 : xbsIndex_r4/Constant  const=10  gui_display_data_type=Fixed-point  arith_type=Unsigned  n_bits=5  bin_pt=0  preci_type=Single  exp_width=8  frac_width=24  explicit_period=off  period=1  equ=P=C  opselect=C  inp2=PCIN>>17  opr=+  inp1=P  carry=CIN  dbl_ovrd=off  block_type=constant
  Constant11 : xbsIndex_r4/Constant  const=11  gui_display_data_type=Fixed-point  arith_type=Unsigned  n_bits=5  bin_pt=0  preci_type=Single  exp_width=8  frac_width=24  explicit_period=off  period=1  equ=P=C  opselect=C  inp2=PCIN>>17  opr=+  inp1=P  carry=CIN  dbl_ovrd=off  block_type=constant
  Constant12 : xbsIndex_r4/Constant  const=12  gui_display_data_type=Fixed-point  arith_type=Unsigned  n_bits=5  bin_pt=0  preci_type=Single  exp_width=8  frac_width=24  explicit_period=off  period=1  equ=P=C  opselect=C  inp2=PCIN>>17  opr=+  inp1=P  carry=CIN  dbl_ovrd=off  block_type=constant
  Constant13 : xbsIndex_r4/Constant  const=13  gui_display_data_type=Fixed-point  arith_type=Unsigned  n_bits=5  bin_pt=0  preci_type=Single  exp_width=8  frac_width=24  explicit_period=off  period=1  equ=P=C  opselect=C  inp2=PCIN>>17  opr=+  inp1=P  carry=CIN  dbl_ovrd=off  block_type=constant
  Constant14 : xbsIndex_r4/Constant  const=14  gui_display_data_type=Fixed-point  arith_type=Unsigned  n_bits=5  bin_pt=0  preci_type=Single  exp_width=8  frac_width=24  explicit_period=off  period=1  equ=P=C  opselect=C  inp2=PCIN>>17  opr=+  inp1=P  carry=CIN  dbl_ovrd=off  block_type=constant
  Constant15 : xbsIndex_r4/Constant  const=15  gui_display_data_type=Fixed-point  arith_type=Unsigned  n_bits=5  bin_pt=0  preci_type=Single  exp_width=8  frac_width=24  explicit_period=off  period=1  equ=P=C  opselect=C  inp2=PCIN>>17  opr=+  inp1=P  carry=CIN  dbl_ovrd=off  block_type=constant
  Constant2 : xbsIndex_r4/Constant  const=2  gui_display_data_type=Fixed-point  arith_type=Unsigned  n_bits=5  bin_pt=0  preci_type=Single  exp_width=8  frac_width=24  explicit_period=off  period=1  equ=P=C  opselect=C  inp2=PCIN>>17  opr=+  inp1=P  carry=CIN  dbl_ovrd=off  block_type=constant
  Constant20 : xbsIndex_r4/Constant  const=31  gui_display_data_type=Fixed-point  arith_type=Unsigned  n_bits=5  bin_pt=0  preci_type=Single  exp_width=8  frac_width=24  explicit_period=off  period=1  equ=P=C  opselect=C  inp2=PCIN>>17  opr=+  inp1=P  carry=CIN  dbl_ovrd=off  block_type=constant
  Constant3 : xbsIndex_r4/Constant  const=3  gui_display_data_type=Fixed-point  arith_type=Unsigned  n_bits=5  bin_pt=0  preci_type=Single  exp_width=8  frac_width=24  explicit_period=off  period=1  equ=P=C  opselect=C  inp2=PCIN>>17  opr=+  inp1=P  carry=CIN  dbl_ovrd=off  block_type=constant
  Constant4 : xbsIndex_r4/Constant  const=4  gui_display_data_type=Fixed-point  arith_type=Unsigned  n_bits=5  bin_pt=0  preci_type=Single  exp_width=8  frac_width=24  explicit_period=off  period=1  equ=P=C  opselect=C  inp2=PCIN>>17  opr=+  inp1=P  carry=CIN  dbl_ovrd=off  block_type=constant
  Constant5 : xbsIndex_r4/Constant  const=5  gui_display_data_type=Fixed-point  arith_type=Unsigned  n_bits=5  bin_pt=0  preci_type=Single  exp_width=8  frac_width=24  explicit_period=off  period=1  equ=P=C  opselect=C  inp2=PCIN>>17  opr=+  inp1=P  carry=CIN  dbl_ovrd=off  block_type=constant
  Constant6 : xbsIndex_r4/Constant  const=6  gui_display_data_type=Fixed-point  arith_type=Unsigned  n_bits=5  bin_pt=0  preci_type=Single  exp_width=8  frac_width=24  explicit_period=off  period=1  equ=P=C  opselect=C  inp2=PCIN>>17  opr=+  inp1=P  carry=CIN  dbl_ovrd=off  block_type=constant
  Constant7 : xbsIndex_r4/Constant  const=7  gui_display_data_type=Fixed-point  arith_type=Unsigned  n_bits=5  bin_pt=0  preci_type=Single  exp_width=8  frac_width=24  explicit_period=off  period=1  equ=P=C  opselect=C  inp2=PCIN>>17  opr=+  inp1=P  carry=CIN  dbl_ovrd=off  block_type=constant
  Constant8 : xbsIndex_r4/Constant  const=8  gui_display_data_type=Fixed-point  arith_type=Unsigned  n_bits=5  bin_pt=0  preci_type=Single  exp_width=8  frac_width=24  explicit_period=off  period=1  equ=P=C  opselect=C  inp2=PCIN>>17  opr=+  inp1=P  carry=CIN  dbl_ovrd=off  block_type=constant
  Constant9 : xbsIndex_r4/Constant  const=9  gui_display_data_type=Fixed-point  arith_type=Unsigned  n_bits=5  bin_pt=0  preci_type=Single  exp_width=8  frac_width=24  explicit_period=off  period=1  equ=P=C  opselect=C  inp2=PCIN>>17  opr=+  inp1=P  carry=CIN  dbl_ovrd=off  block_type=constant
  Counter : xbsIndex_r4/Counter  cnt_type=Count Limited  cnt_to=31  operation=Up  start_count=0  cnt_by_val=1  arith_type=Unsigned  n_bits=5  bin_pt=0  load_pin=off  rst=on  en=on  explicit_period=off  period=Tclk  use_behavioral_HDL=off  implementation=Fabric  dbl_ovrd=off  block_type=counter
  DAC Sum1 : Subsystem
  DC_decimate : Subsystem
  Delay : xbsIndex_r4/Delay  rst=off  infoeditControl=Selection of Reset will increase slice count due to use of real FFs and instead of SRLs  en=off  latency=6  reg_retiming=off  dbl_ovrd=off  block_type=delay
  Demux : Demux  Outputs=2
  Demux1 : Demux  Outputs=2
  Gateway Out{1,7..10,23} (6 alike) : xbsIndex_r4/Gateway Out  inherit_from_input=off  hdl_port=off  rows=1  columns=1  UseAsDAC=off  DACChannel='1'  interface=None  automatic_assignment=on  address_offset=hex2dec('00')  intf_name=''  intf_description=''  timing_constraint=None  locs_specified=off  LOCs={}  io_standard={}  block_type=gatewayout
  Mux{,1,6..7} (4 alike) : Mux  Inputs=2
  Mux16X4 : Subsystem
  Relational : xbsIndex_r4/Relational  mode=a!=b  op_type=Bool  en=off  latency=0  dbl_ovrd=off  block_type=relational
  debug Scope : Subsystem
  oneLineUpDown0 : Subsystem
  oneLineUpDown1 : Subsystem
  oneLineUpDown10 : Subsystem
  oneLineUpDown11 : Subsystem
  oneLineUpDown12 : Subsystem
  oneLineUpDown13 : Subsystem
  oneLineUpDown14 : Subsystem
  oneLineUpDown15 : Subsystem
  oneLineUpDown2 : Subsystem
  oneLineUpDown3 : Subsystem
  oneLineUpDown4 : Subsystem
  oneLineUpDown5 : Subsystem
  oneLineUpDown6 : Subsystem
  oneLineUpDown7 : Subsystem
  oneLineUpDown8 : Subsystem
  oneLineUpDown9 : Subsystem
  synch scope : Scope  NumInputPorts=2
  toDAC : Outport
  demodulated : Outport  Port=2
  wires:
  [fpgaReset] -> Counter/1, Delay/1
  Gateway Out10/1 -> Mux7/2
  Gateway Out9/1 -> Mux7/1
  Gateway Out8/1 -> Mux6/2
  Gateway Out7/1 -> Mux6/1
  Mux6/1 -> BDC scope/1
  Mux7/1 -> BDC scope/2
  Demux/1 -> Gateway Out7/1
  Demux1/2 -> Gateway Out10/1
  Demux1/1 -> Gateway Out9/1
  Demux/2 -> Gateway Out8/1
  Delay/1 -> Mux16X4/1(synch)
  Constant/1 -> oneLineUpDown0/2(addrIn)
  Counter/1 -> Gateway Out23/1, oneLineUpDown1/3(synchIn), oneLineUpDown2/3(synchIn), oneLineUpDown3/3(synchIn), oneLineUpDown4/3(synchIn), oneLineUpDown5/3(synchIn), oneLineUpDown6/3(synchIn), oneLineUpDown7/3(synchIn), oneLineUpDown8/3(synchIn), oneLineUpDown9/3(synchIn), oneLineUpDown10/3(synchIn), oneLineUpDown11/3(synchIn), oneLineUpDown12/3(synchIn), oneLineUpDown13/3(synchIn), oneLineUpDown15/3(synchIn), oneLineUpDown14/3(synchIn), oneLineUpDown0/3(synchIn), Relational/2
  Gateway Out23/1 -> synch scope/1
  Gateway Out1/1 -> synch scope/2
  Relational/1 -> Gateway Out1/1, Counter/2
  Constant20/1 -> Relational/1
  oneLineUpDown0/1(DC_Out) -> debug Scope/1(demod), Mux16X4/2(line0)  "DC_out_line0"
  oneLineUpDown1/1(DC_Out) -> Mux16X4/3(line1)  "DC_out_line1"
  oneLineUpDown2/1(DC_Out) -> Mux16X4/4(line2)  "DC_out_line2"
  oneLineUpDown3/1(DC_Out) -> Mux16X4/5(line3)  "DC_out_line3"
  oneLineUpDown4/1(DC_Out) -> Mux16X4/6(line4)  "DC_out_line4"
  oneLineUpDown5/1(DC_Out) -> Mux16X4/7(line5)  "DC_out_line5"
  oneLineUpDown6/1(DC_Out) -> Mux16X4/8(line6)  "DC_out_line6"
  oneLineUpDown7/1(DC_Out) -> Mux16X4/9(line7)  "DC_out_line7"
  oneLineUpDown8/1(DC_Out) -> Mux16X4/10(line8)  "DC_out_line8"
  oneLineUpDown9/1(DC_Out) -> Mux16X4/11(line9)  "DC_out_line9"
  oneLineUpDown10/1(DC_Out) -> Mux16X4/12(line10)  "DC_out_line10"
  oneLineUpDown11/1(DC_Out) -> Mux16X4/13(line11)  "DC_out_line11"
  oneLineUpDown12/1(DC_Out) -> Mux16X4/14(line12)  "DC_out_line12"
  oneLineUpDown13/1(DC_Out) -> Mux16X4/15(line13)  "DC_out_line13"
  oneLineUpDown14/1(DC_Out) -> Mux16X4/16(line14)  "DC_out_line14"
  oneLineUpDown15/1(DC_Out) -> Mux16X4/17(line15)  "DC_out_line15"
  oneLineUpDown15/2(UC_out) -> DAC Sum1/1(In1)  "UC_out_line15"
  oneLineUpDown14/2(UC_out) -> DAC Sum1/2(In2)  "UC_out_line14"
  oneLineUpDown13/2(UC_out) -> DAC Sum1/3(In3)  "UC_out_line13"
  oneLineUpDown12/2(UC_out) -> DAC Sum1/4(In4)  "UC_out_line12"
  oneLineUpDown11/2(UC_out) -> DAC Sum1/5(In5)  "UC_out_line11"
  oneLineUpDown10/2(UC_out) -> DAC Sum1/6(In6)  "UC_out_line10"
  oneLineUpDown9/2(UC_out) -> DAC Sum1/7(In7)  "UC_out_line9"
  oneLineUpDown8/2(UC_out) -> DAC Sum1/8(In8)  "UC_out_line8"
  oneLineUpDown7/2(UC_out) -> DAC Sum1/9(In9)  "UC_out_line7"
  oneLineUpDown6/2(UC_out) -> DAC Sum1/10(In10)  "UC_out_line6"
  oneLineUpDown5/2(UC_out) -> DAC Sum1/11(In11)  "UC_out_line5"
  oneLineUpDown4/2(UC_out) -> DAC Sum1/12(In12)  "UC_out_line4"
  oneLineUpDown3/2(UC_out) -> DAC Sum1/13(In13)  "UC_out_line3"
  oneLineUpDown2/2(UC_out) -> DAC Sum1/14(In14)  "UC_out_line2"
  oneLineUpDown1/2(UC_out) -> DAC Sum1/15(In15)  "UC_out_line1"
  oneLineUpDown0/3(UC_out) -> DAC Sum1/16(In16)  "UC_out_line0"
  Constant1/1 -> oneLineUpDown1/2(addrIn)
  Constant2/1 -> oneLineUpDown2/2(addrIn)
  Constant3/1 -> oneLineUpDown3/2(addrIn)
  Constant4/1 -> oneLineUpDown4/2(addrIn)
  Constant5/1 -> oneLineUpDown5/2(addrIn)
  Constant6/1 -> oneLineUpDown6/2(addrIn)
  Constant7/1 -> oneLineUpDown7/2(addrIn)
  Constant8/1 -> oneLineUpDown8/2(addrIn)
  Constant9/1 -> oneLineUpDown9/2(addrIn)
  Constant10/1 -> oneLineUpDown10/2(addrIn)
  Constant11/1 -> oneLineUpDown11/2(addrIn)
  Constant12/1 -> oneLineUpDown12/2(addrIn)
  Constant13/1 -> oneLineUpDown13/2(addrIn)
  Constant14/1 -> oneLineUpDown14/2(addrIn)
  Constant15/1 -> oneLineUpDown15/2(addrIn)
  ADC_Q_in/1 -> Mux/1
  ADC_I_in/1 -> Mux/2
  REF_Q_in1/1 -> Mux1/2
  REF_I_in1/1 -> Mux1/1
  Mux/1 -> oneLineUpDown1/1(ADC_IQ_in), oneLineUpDown2/1(ADC_IQ_in), Demux/1, oneLineUpDown3/1(ADC_IQ_in), oneLineUpDown4/1(ADC_IQ_in), oneLineUpDown5/1(ADC_IQ_in), oneLineUpDown6/1(ADC_IQ_in), oneLineUpDown7/1(ADC_IQ_in), oneLineUpDown8/1(ADC_IQ_in), oneLineUpDown9/1(ADC_IQ_in), oneLineUpDown10/1(ADC_IQ_in), oneLineUpDown11/1(ADC_IQ_in), oneLineUpDown12/1(ADC_IQ_in), oneLineUpDown13/1(ADC_IQ_in), oneLineUpDown15/1(ADC_IQ_in), oneLineUpDown14/1(ADC_IQ_in), oneLineUpDown0/1(ADC_IQ_in)
  Mux1/1 -> oneLineUpDown0/4(REF_IQ_in1), oneLineUpDown1/4(REF_IQ_in1), oneLineUpDown2/4(REF_IQ_in1), oneLineUpDown3/4(REF_IQ_in1), oneLineUpDown4/4(REF_IQ_in1), Demux1/1, oneLineUpDown5/4(REF_IQ_in1), oneLineUpDown6/4(REF_IQ_in1), oneLineUpDown7/4(REF_IQ_in1), oneLineUpDown8/4(REF_IQ_in1), oneLineUpDown9/4(REF_IQ_in1), oneLineUpDown10/4(REF_IQ_in1), oneLineUpDown11/4(REF_IQ_in1), oneLineUpDown12/4(REF_IQ_in1), oneLineUpDown13/4(REF_IQ_in1), oneLineUpDown15/4(REF_IQ_in1), oneLineUpDown14/4(REF_IQ_in1)
  DAC Sum1/1(Out1) -> toDAC/1
  Mux16X4/1(Out1) -> DC_decimate/1(In1)
  DC_decimate/1(dec_sig_ref) -> demodulated/1
  oneLineUpDown0/2(Freq) -> debug Scope/2(freq)
